simulink model "Model"  (R2026a)
settings: Solver=VariableStepAuto  StopTime=t_total(end)
values from neighbouring files (symbols this model uses):
  Beat = 1    [Ld_Identification_m.m]    (also in Lq_Identification_m.m)
  J = 0.00062    [Ld_Identification_m.m]    (also in Lq_Identification_m.m)
  Ld = 2e-3    (= 0.002)    [Ld_Identification_m.m]    (also in Lq_Identification_m.m)
  Lq = 2.5e-3    (= 0.0025)    [Ld_Identification_m.m]    (also in Lq_Identification_m.m)
  np = 14    [Ld_Identification_m.m]    (also in Lq_Identification_m.m)
  Switch = -1    [Ld_Identification_m.m]    (also in Lq_Identification_m.m = 1)
  Ts = 1/f    (= 6.66666666667e-05)    [Ld_Identification_m.m]    (also in Lq_Identification_m.m)
  Udc = 12    [Ld_Identification_m.m]    (also in Lq_Identification_m.m)
libraries: sl_discontinuities x6, simulink x3, autolibpmsminterior x1
settings Model: Creator=mushen  LastModifiedBy=mushen

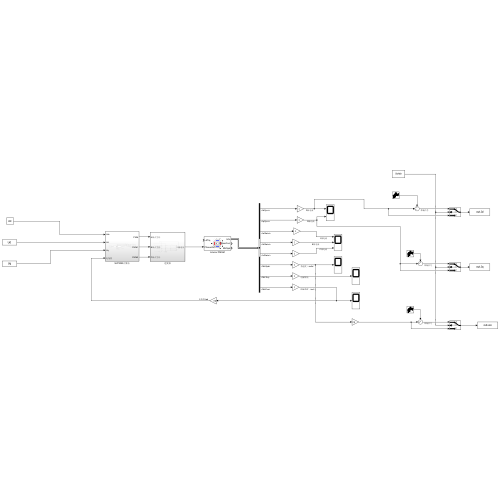
[thumbnail: Simulink's stored preview of the top-level diagram]
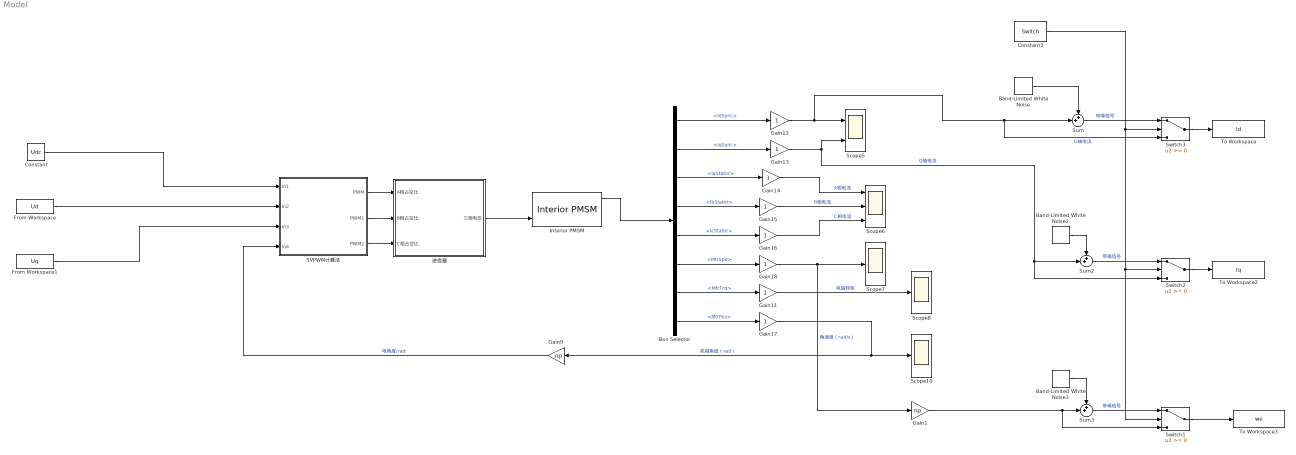
== system Model ==
  Band-Limited White Noise : simulink/Sources/Band-Limited White Noise  Cov=[0.000000005]  Ts=Ts  seed=100
  Band-Limited White Noise2 : simulink/Sources/Band-Limited White Noise  Cov=[0.000000005]  Ts=Ts  seed=100
  Band-Limited White Noise3 : simulink/Sources/Band-Limited White Noise  Cov=[0.00001]  Ts=Ts  seed=100
  Bus Selector : BusSelector  OutputSignals=IdSync,IqSync,IaStator,IbStator,IcStator,MtrSpd,MtrTrq,MtrPos
  Constant : Constant  Value=Udc
  Constant2 : Constant  Value=Switch  VectorParams1D=off
  From Workspace : FromWorkspace  VariableName=Ud
  From Workspace1 : FromWorkspace  VariableName=Uq
  Gain1 : Gain  Gain=np
  Gain{11..18} (8 alike) : Gain
  Gain9 : Gain  Gain=np
  Interior PMSM : autolibpmsminterior/Interior PMSM  port_config=Torque  sim_type=Continuous  Ts=0.001  P=np  Rs=Rs  Ldq=[Ld Lq]  KConstText=Permanent flux linkage constant (lambda_pm):  lambda_pm=Psi  Ke=159.9771  mechanical=[J,4.924e-4,0]  idq0=[0 0]  theta_init=0  omega_init=0  KConst=0.2205  lambda_pm_calc=0.2205  Kt=0.07  RefBlkName='autolibpmsminterior/Interior PMSM'  aMode=5
      settings: LibrarySourceBlock=mcblib/Electrical Systems/Motors/Interior PMSM
  SVPWM计算法 : Subsystem
  Scope10 : Scope
      settings: ActiveDisplayYMinimum=-6.5677946015674407E-40  ActiveDisplayYMaximum=4.8046153207722005E-20  DataLoggingVariableName=ScopeData13
  Scope5 : Scope  NumInputPorts=2
      settings: ActiveDisplayYMinimum=-1  ActiveDisplayYMaximum=1  DataLoggingVariableName=ScopeData12
  Scope6 : Scope  NumInputPorts=3
      settings: ActiveDisplayYMinimum=-0.86567841566342707  ActiveDisplayYMaximum=0.50118224064724726  DataLoggingVariableName=ScopeData14
  Scope7 : Scope
      settings: ActiveDisplayYMinimum=-8.3500269440904287  ActiveDisplayYMaximum=20.77178175547505  DataLoggingVariableName=ScopeData10
  Scope8 : Scope
      settings: ActiveDisplayYMinimum=-5.4423436911446466E-14  ActiveDisplayYMaximum=6.0470485460760218E-15  DataLoggingVariableName=ScopeData11
  Sum : Sum  Inputs=++|
  Sum2 : Sum  Inputs=++|
  Sum3 : Sum  Inputs=++|
  Switch1 : Switch  SaturateOnIntegerOverflow=off  InputSameDT=off
  Switch2 : Switch  SaturateOnIntegerOverflow=off  InputSameDT=off
  Switch3 : Switch  SaturateOnIntegerOverflow=off  InputSameDT=off
  To Workspace : ToWorkspace  VariableName=Id  SaveFormat=Timeseries  SampleTime=Ts
  To Workspace2 : ToWorkspace  VariableName=Iq  SaveFormat=Timeseries  SampleTime=Ts
  To Workspace3 : ToWorkspace  VariableName=we  SaveFormat=Timeseries  SampleTime=Ts
  逆变器 : Subsystem
  wires:
  From Workspace1/1 -> SVPWM计算法/3(In3)
  Constant/1 -> SVPWM计算法/1(In1)
  SVPWM计算法/1(PWM) -> 逆变器/1(A相占空比)
  Gain9/1 -> SVPWM计算法/4(In4)  "电角度/rad"
  From Workspace/1 -> SVPWM计算法/2(In2)
  Band-Limited White Noise/1 -> Sum/1
  SVPWM计算法/2(PWM1) -> 逆变器/2(B相占空比)
  Sum/1 -> Switch3/1  "带噪信号"
  SVPWM计算法/3(PWM2) -> 逆变器/3(C相占空比)
  Bus Selector/4 -> Gain15/1  "<IbStator>"
  Gain13/1 -> Scope5/2, Switch2/3, Sum2/2  "Q轴电流"
  Bus Selector/3 -> Gain14/1  "<IaStator>"
  Gain18/1 -> Gain1/1, Scope7/1  "角速度（rad/s）"
  Bus Selector/6 -> Gain18/1  "<MtrSpd>"
  Bus Selector/7 -> Gain11/1  "<MtrTrq>"
  Bus Selector/5 -> Gain16/1  "<IcStator>"
  Interior PMSM/1 -> Bus Selector/1
  Bus Selector/1 -> Gain12/1  "<IdSync>"
  Gain11/1 -> Scope8/1  "电磁转矩"
  Gain17/1 -> Gain9/1, Scope10/1  "机械角度（rad）"
  Gain15/1 -> Scope6/2  "B相电流"
  Gain14/1 -> Scope6/1  "A相电流"
  Gain16/1 -> Scope6/3  "C相电流"
  Bus Selector/2 -> Gain13/1  "<IqSync>"
  Bus Selector/8 -> Gain17/1  "<MtrPos>"
  Gain12/1 -> Switch3/3, Sum/2, Scope5/1  "D轴电流"
  逆变器/1(三相电压) -> Interior PMSM/2
  Switch3/1 -> To Workspace/1
  Constant2/1 -> Switch1/2, Switch2/2, Switch3/2
  Sum2/1 -> Switch2/1  "带噪信号"
  Band-Limited White Noise2/1 -> Sum2/1
  Switch1/1 -> To Workspace3/1
  Band-Limited White Noise3/1 -> Sum3/1
  Sum3/1 -> Switch1/1  "带噪信号"
  Gain1/1 -> Switch1/3, Sum3/2
  Switch2/1 -> To Workspace2/1

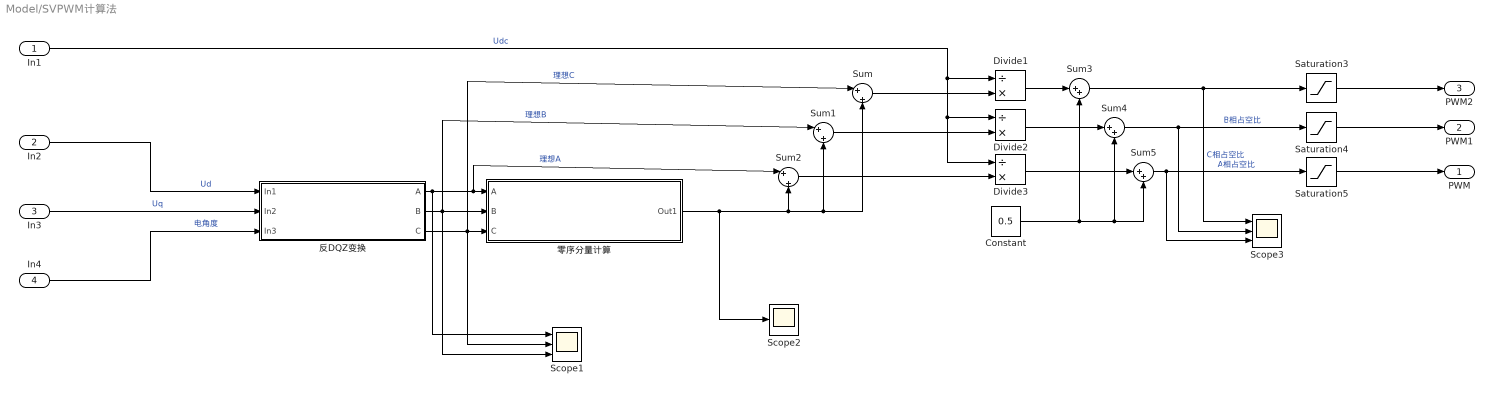
== system Model/SVPWM计算法 ==
  In1 : Inport
  In2 : Inport  Port=2
  In3 : Inport  Port=3
  In4 : Inport  Port=4
  Constant : Constant  Value=0.5
  Divide1 : Product  Inputs=/*
  Divide2 : Product  Inputs=/*
  Divide3 : Product  Inputs=/*
  Saturation3 : Saturate  UpperLimit=1  LowerLimit=0
  Saturation4 : Saturate  UpperLimit=1  LowerLimit=0
  Saturation5 : Saturate  UpperLimit=1  LowerLimit=0
  Scope1 : Scope  NumInputPorts=3
      settings: ActiveDisplayYMinimum=-3.13505  ActiveDisplayYMaximum=3.34432  DataLoggingVariableName=ScopeData2
  Scope2 : Scope
      settings: ActiveDisplayYMinimum=-0.20463  ActiveDisplayYMaximum=-0.00463  DataLoggingVariableName=ScopeData4
  Scope3 : Scope  NumInputPorts=3
      settings: ActiveDisplayYMinimum=0.0625  ActiveDisplayYMaximum=0.9375  DataLoggingVariableName=ScopeData3
  Sum : Sum  Inputs=|+|+
  Sum1 : Sum  Inputs=|+|+
  Sum2 : Sum  Inputs=|+|+
  Sum3 : Sum  Inputs=|++
  Sum4 : Sum  Inputs=|++
  Sum5 : Sum  Inputs=|++
  反DQZ变换 : Subsystem
  零序分量计算 : Subsystem
  PWM : Outport
  PWM1 : Outport  Port=2
  PWM2 : Outport  Port=3
  wires:
  Sum5/1 -> Scope3/3, Saturation5/1  "A相占空比"
  Sum4/1 -> Saturation4/1, Scope3/2  "B相占空比"
  In3/1 -> 反DQZ变换/2(In2)  "Uq"
  In4/1 -> 反DQZ变换/3(In3)  "电角度"
  Sum3/1 -> Scope3/1, Saturation3/1  "C相占空比"
  In2/1 -> 反DQZ变换/1(In1)  "Ud"
  反DQZ变换/1(A) -> Sum2/1, 零序分量计算/1(A), Scope1/1  "理想A"
  反DQZ变换/2(B) -> Sum1/1, Scope1/3, 零序分量计算/2(B)  "理想B"
  反DQZ变换/3(C) -> Sum/1, Scope1/2, 零序分量计算/3(C)  "理想C"
  零序分量计算/1(Out1) -> Sum2/2, Sum/2, Sum1/2, Scope2/1
  Sum2/1 -> Divide3/2
  Sum1/1 -> Divide2/2
  Sum/1 -> Divide1/2
  In1/1 -> Divide3/1, Divide2/1, Divide1/1  "Udc"
  Divide1/1 -> Sum3/1
  Divide3/1 -> Sum5/1
  Divide2/1 -> Sum4/1
  Constant/1 -> Sum3/2, Sum4/2, Sum5/2
  Saturation4/1 -> PWM1/1
  Saturation3/1 -> PWM2/1
  Saturation5/1 -> PWM/1

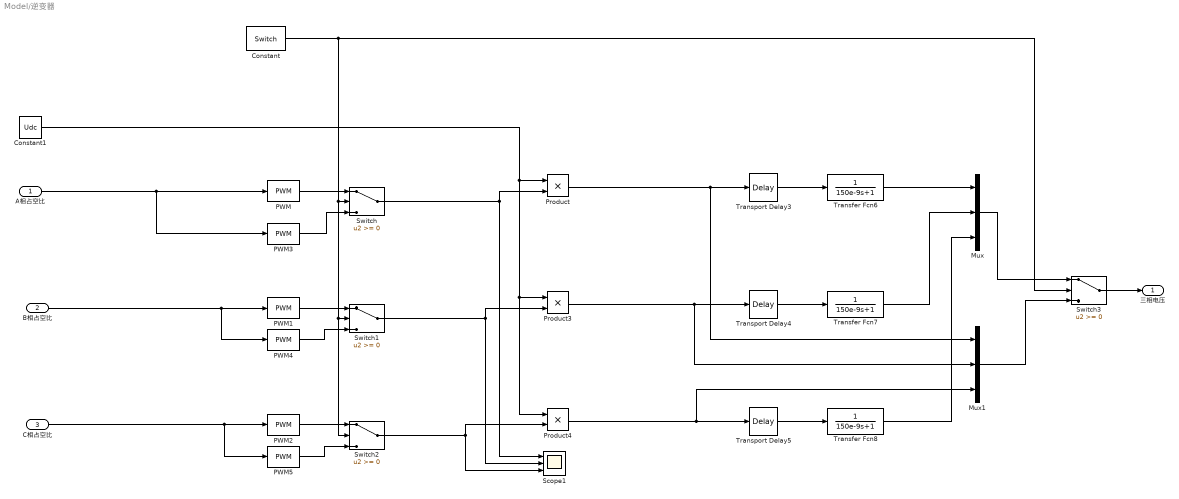
== system Model/逆变器 ==
  A相占空比 : Inport
  B相占空比 : Inport  Port=2
  C相占空比 : Inport  Port=3
  Constant : Constant  Value=Switch  VectorParams1D=off
  Constant1 : Constant  Value=Udc
  Mux : Mux  Inputs=3
  Mux1 : Mux  Inputs=3
  PWM : sl_discontinuities/PWM  DisableCoverage=on  Period=Ts  InitialDelay=Beat*Ts  DisallowZeroDutyCycle=off  RunAtFixedTimeIntervals=off  SampleTime=Ts
  PWM1 : sl_discontinuities/PWM  DisableCoverage=on  Period=Ts  InitialDelay=Beat*Ts  DisallowZeroDutyCycle=off  RunAtFixedTimeIntervals=off  SampleTime=Ts
  PWM2 : sl_discontinuities/PWM  DisableCoverage=on  Period=Ts  InitialDelay=Beat*Ts  DisallowZeroDutyCycle=off  RunAtFixedTimeIntervals=off  SampleTime=Ts
  PWM3 : sl_discontinuities/PWM  DisableCoverage=on  Period=Ts  InitialDelay=0  DisallowZeroDutyCycle=off  RunAtFixedTimeIntervals=off  SampleTime=Ts
  PWM4 : sl_discontinuities/PWM  DisableCoverage=on  Period=Ts  InitialDelay=0  DisallowZeroDutyCycle=off  RunAtFixedTimeIntervals=off  SampleTime=Ts
  PWM5 : sl_discontinuities/PWM  DisableCoverage=on  Period=Ts  InitialDelay=0  DisallowZeroDutyCycle=off  RunAtFixedTimeIntervals=off  SampleTime=Ts
  Product : Product
  Product3 : Product
  Product4 : Product
  Scope1 : Scope  NumInputPorts=3
      settings: ActiveDisplayYMinimum=-0.125  ActiveDisplayYMaximum=1.125
  Switch{,1..3} (4 alike) : Switch  SaturateOnIntegerOverflow=off  InputSameDT=off
  Transfer Fcn6 : TransferFcn  Denominator=[150e-9 1]
  Transfer Fcn7 : TransferFcn  Denominator=[150e-9 1]
  Transfer Fcn8 : TransferFcn  Denominator=[150e-9 1]
  Transport Delay3 : TransportDelay  DelayTime=0.5e-6  TransDelayFeedthrough=on  PadeOrder=1
  Transport Delay4 : TransportDelay  DelayTime=0.5e-6  TransDelayFeedthrough=on  PadeOrder=1
  Transport Delay5 : TransportDelay  DelayTime=0.5e-6  TransDelayFeedthrough=on  PadeOrder=1
  三相电压 : Outport
  wires:
  Constant1/1 -> Product4/1, Product3/1, Product/1
  Transport Delay3/1 -> Transfer Fcn6/1
  Product/1 -> Mux1/1, Transport Delay3/1
  Transport Delay4/1 -> Transfer Fcn7/1
  Transport Delay5/1 -> Transfer Fcn8/1
  Product4/1 -> Mux1/3, Transport Delay5/1
  Product3/1 -> Mux1/2, Transport Delay4/1
  A相占空比/1 -> PWM3/1, PWM/1
  B相占空比/1 -> PWM4/1, PWM1/1
  C相占空比/1 -> PWM5/1, PWM2/1
  PWM/1 -> Switch/1
  PWM3/1 -> Switch/3
  Switch/1 -> Product/2, Scope1/1
  PWM1/1 -> Switch1/1
  PWM4/1 -> Switch1/3
  Switch1/1 -> Product3/2, Scope1/2
  PWM2/1 -> Switch2/1
  PWM5/1 -> Switch2/3
  Switch2/1 -> Scope1/3, Product4/2
  Mux/1 -> Switch3/1
  Transfer Fcn6/1 -> Mux/1
  Transfer Fcn7/1 -> Mux/2
  Transfer Fcn8/1 -> Mux/3
  Mux1/1 -> Switch3/3
  Switch3/1 -> 三相电压/1
  Constant/1 -> Switch3/2, Switch/2, Switch2/2, Switch1/2

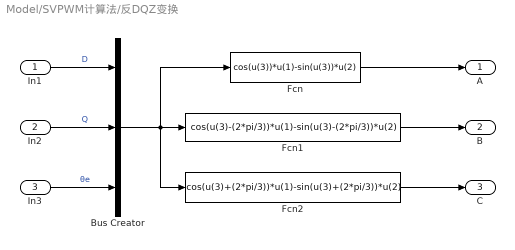
== system Model/SVPWM计算法/反DQZ变换 ==
  In1 : Inport
  In2 : Inport  Port=2
  In3 : Inport  Port=3
  Bus Creator : BusCreator  Inputs=3
  Fcn : Fcn  Expr=cos(u(3))*u(1)-sin(u(3))*u(2)
  Fcn1 : Fcn  Expr=cos(u(3)-(2*pi/3))*u(1)-sin(u(3)-(2*pi/3))*u(2)
  Fcn2 : Fcn  Expr=cos(u(3)+(2*pi/3))*u(1)-sin(u(3)+(2*pi/3))*u(2)
  A : Outport
  B : Outport  Port=2
  C : Outport  Port=3
  wires:
  In3/1 -> Bus Creator/3  "θe"
  In2/1 -> Bus Creator/2  "Q"
  In1/1 -> Bus Creator/1  "D"
  Bus Creator/1 -> Fcn/1, Fcn1/1, Fcn2/1
  Fcn/1 -> A/1
  Fcn1/1 -> B/1
  Fcn2/1 -> C/1

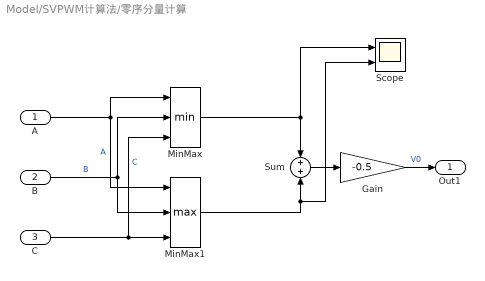
== system Model/SVPWM计算法/零序分量计算 ==
  A : Inport
  B : Inport  Port=2
  C : Inport  Port=3
  Gain : Gain  Gain=-0.5
  MinMax : MinMax  Inputs=3
  MinMax1 : MinMax  Function=max  Inputs=3
  Scope : Scope  NumInputPorts=2
      settings: ActiveDisplayYMinimum=-3.75  ActiveDisplayYMaximum=3.75  DataLoggingVariableName=ScopeData3
  Sum : Sum
  Out1 : Outport
  wires:
  A/1 -> MinMax/1, MinMax1/1  "A"
  B/1 -> MinMax1/2, MinMax/2  "B"
  C/1 -> MinMax/3, MinMax1/3  "C"
  MinMax/1 -> Sum/1, Scope/1
  MinMax1/1 -> Scope/2, Sum/2
  Sum/1 -> Gain/1
  Gain/1 -> Out1/1  "V0"
